simulink subsystem "FlightControl"  (R2024b)
settings: Solver=VariableStepAuto  StartTime=0.0  StopTime=10.0  RelTol=1e-3
undefined symbols (not defined in the file): control, controlParams, ControlSampleTime, CriticalTiltAngle, DiscIntNeverNeededParam, flightState, FWControlParams, FWTrimSpeed, tilt_max, tilt_trim, TiltScheduleRate, uavParam, w_trim, WindDownRate
libraries: slpidlib x31, simulink x9
(part 1 of 5)
settings Model: Creator=jjha  LastModifiedBy=jjha

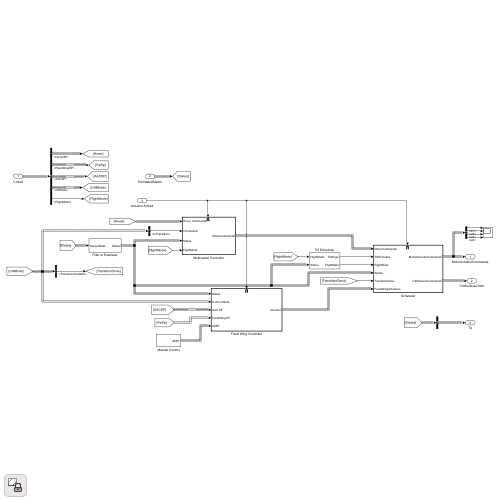
[thumbnail: Simulink's stored preview of the top-level diagram]
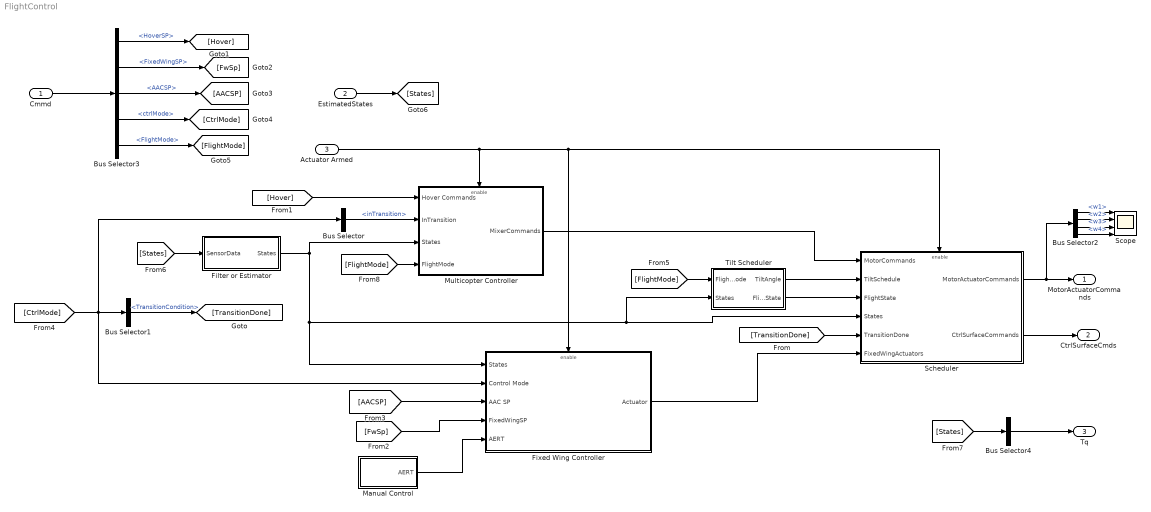
== system FlightControl ==
  Cmmd : Inport
  EstimatedStates : Inport  Port=2
  Actuator Armed : Inport  Port=3
  Bus Selector : BusSelector  OutputSignals=inTransition
  Bus Selector1 : BusSelector  OutputSignals=TransitionCondition
  Bus Selector2 : BusSelector  OutputSignals=w1,w2,w3,w4
  Bus Selector3 : BusSelector  OutputSignals=HoverSP,FixedWingSP,AACSP,ctrlMode,FlightMode
  Bus Selector4 : BusSelector  OutputSignals=RotorParameters.T1,RotorParameters.T2,RotorParameters.T3,RotorParameters.T4  OutputAsBus=on
  Filter or Estimator : Subsystem
  Fixed Wing Controller : Subsystem  TreatAsAtomicUnit=on  VariantControl=Fixed Wing Controller
  Manual Control : Subsystem
  Multicopter Controller : Subsystem
  Scheduler : Subsystem  SystemSampleTime=0.005
  Scope : Scope  NumInputPorts=4
  Tilt Scheduler : Subsystem
  MotorActuatorCommands : Outport
  CtrlSurfaceCmds : Outport  Port=2
  Tq : Outport  Port=3
  wires:
  Bus Selector3/2 -> [FwSp]  "<FixedWingSP>"
  Bus Selector3/1 -> [Hover]  "<HoverSP>"
  Bus Selector1/1 -> [TransitionDone]  "<TransitionCondition>"
  [Hover] -> Multicopter Controller/1(Hover Commands)
  Cmmd/1 -> Bus Selector3/1
  Bus Selector3/3 -> [AACSP]  "<AACSP>"
  Bus Selector2/4 -> Scope/4  "<w4>"
  Bus Selector3/5 -> [FlightMode]  "<FlightMode>"
  [FlightMode] -> Tilt Scheduler/1(FlightMode)
  [States] -> Bus Selector4/1
  Manual Control/1(AERT) -> Fixed Wing Controller/5(AERT)
  Tilt Scheduler/2(FlightState) -> Scheduler/3(FlightState)
  [AACSP] -> Fixed Wing Controller/3(AAC SP)
  Bus Selector3/4 -> [CtrlMode]  "<ctrlMode>"
  Multicopter Controller/1(MixerCommands) -> Scheduler/1(MotorCommands)
  Scheduler/2(CtrlSurfaceCommands) -> CtrlSurfaceCmds/1
  [CtrlMode] -> Bus Selector/1, Bus Selector1/1, Fixed Wing Controller/2(Control Mode)
  Bus Selector2/3 -> Scope/3  "<w3>"
  [FwSp] -> Fixed Wing Controller/4(FixedWingSP)
  [TransitionDone] -> Scheduler/5(TransitionDone)
  EstimatedStates/1 -> [States]
  Filter or Estimator/1(States) -> Tilt Scheduler/2(States), Scheduler/4(States), Fixed Wing Controller/1(States), Multicopter Controller/3(States)
  Bus Selector/1 -> Multicopter Controller/2(InTransition)  "<inTransition>"
  Tilt Scheduler/1(TiltAngle) -> Scheduler/2(TiltSchedule)
  Scheduler/1(MotorActuatorCommands) -> Bus Selector2/1, MotorActuatorCommands/1
  Bus Selector4/1 -> Tq/1
  [States] -> Filter or Estimator/1(SensorData)
  Fixed Wing Controller/1(Actuator) -> Scheduler/6(FixedWingActuators)
  Bus Selector2/1 -> Scope/1  "<w1>"
  Bus Selector2/2 -> Scope/2  "<w2>"
  [FlightMode] -> Multicopter Controller/4(FlightMode)
  Actuator Armed/1 -> Multicopter Controller/Enable, Scheduler/Enable, Fixed Wing Controller/Enable

== system FlightControl/Filter or Estimator ==
  SensorData : Inport
  States : Outport
  wires:
  SensorData/1 -> States/1

== system FlightControl/Fixed Wing Controller ==
  States : Inport
  Control Mode : Inport  Port=2
  AAC SP : Inport  Port=3
  FixedWingSP : Inport  Port=4
  AERT : Inport  Port=5
  Enable : EnablePort
  Fixed Wing Controller Module : Subsystem  Variant=on  VariantControl=TuningMode == 0
  Actuator : Outport
  wires:
  Fixed Wing Controller Module/1(Actuator) -> Actuator/1
  AERT/1 -> Fixed Wing Controller Module/5(AERT)
  FixedWingSP/1 -> Fixed Wing Controller Module/4(FixedWingSP)
  AAC SP/1 -> Fixed Wing Controller Module/3(AAC SP)
  Control Mode/1 -> Fixed Wing Controller Module/2(Control Mode)
  States/1 -> Fixed Wing Controller Module/1(States)

== system FlightControl/Manual Control ==
  Bus Creator : BusCreator  Inputs=4
  Constant{,1..3} (4 alike) : Constant  Value=0
  AERT : Outport
  wires:
  Constant/1 -> Bus Creator/1  "aileron"
  Constant1/1 -> Bus Creator/2  "throttle"
  Constant2/1 -> Bus Creator/3  "elevator"
  Constant3/1 -> Bus Creator/4  "rudder"
  Bus Creator/1 -> AERT/1

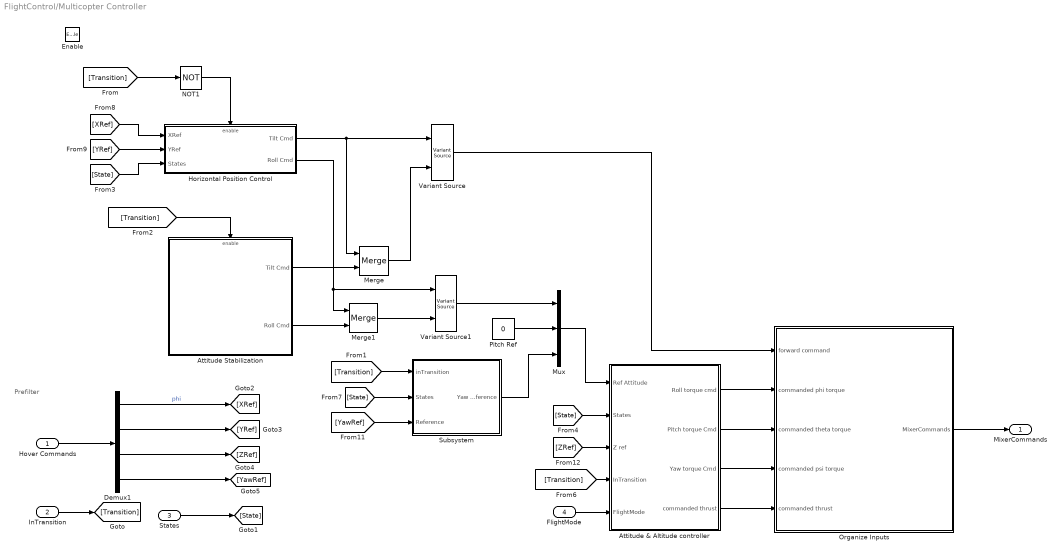
== system FlightControl/Multicopter Controller ==
  note: Prefilter
  Hover Commands : Inport
  InTransition : Inport  Port=2
  States : Inport  Port=3
  FlightMode : Inport  Port=4
  Enable : EnablePort
  Attitude & Altitude controller : Subsystem
  Attitude Stabilization : Subsystem  TreatAsAtomicUnit=on
  Demux1 : Demux
  Horizontal Position Control : Subsystem  TreatAsAtomicUnit=on
  Merge : Merge
  Merge1 : Merge
  Mux : Mux  Inputs=3
  NOT1 : Logic  Operator=NOT  IconShape=distinctive  AllPortsSameDT=off  OutDataTypeStr=boolean
  Organize Inputs : Subsystem
  Pitch Ref : Constant  Value=0
  Subsystem : Subsystem
  Variant Source : VariantSource
  Variant Source1 : VariantSource
  MixerCommands : Outport
  wires:
  Organize Inputs/1(MixerCommands) -> MixerCommands/1
  [Transition] -> Subsystem/1(inTransition)
  [State] -> Subsystem/2(States)
  Attitude Stabilization/2(Roll Cmd) -> Merge1/2
  Variant Source/1 -> Organize Inputs/1(forward command)
  [YawRef] -> Subsystem/3(Reference)
  Merge1/1 -> Variant Source1/2
  Horizontal Position Control/2(Roll Cmd) -> Merge1/1, Variant Source1/1
  Merge/1 -> Variant Source/2
  NOT1/1 -> Horizontal Position Control/Enable
  [Transition] -> Attitude Stabilization/Enable
  Pitch Ref/1 -> Mux/2
  [YRef] -> Horizontal Position Control/2(YRef)
  Attitude Stabilization/1(Tilt Cmd) -> Merge/2
  Demux1/3 -> [ZRef]
  [State] -> Attitude & Altitude controller/2(States)
  FlightMode/1 -> Attitude & Altitude controller/5(FlightMode)
  Attitude & Altitude controller/3(Yaw torque Cmd) -> Organize Inputs/4(commanded psi torque)
  [ZRef] -> Attitude & Altitude controller/3(Z ref)
  [XRef] -> Horizontal Position Control/1(XRef)
  Attitude & Altitude controller/4(commanded thrust) -> Organize Inputs/5(commanded thrust)
  InTransition/1 -> [Transition]
  States/1 -> [State]
  Subsystem/1(Yaw Reference) -> Mux/3
  Demux1/1 -> [XRef]  "phi"
  Attitude & Altitude controller/1(Roll torque cmd) -> Organize Inputs/2(commanded phi torque)
  Attitude & Altitude controller/2(Pitch torque Cmd) -> Organize Inputs/3(commanded theta torque)
  Hover Commands/1 -> Demux1/1
  Demux1/4 -> [YawRef]
  [Transition] -> NOT1/1
  Variant Source1/1 -> Mux/1
  [State] -> Horizontal Position Control/3(States)
  Horizontal Position Control/1(Tilt Cmd) -> Variant Source/1, Merge/1
  Mux/1 -> Attitude & Altitude controller/1(Ref Attitude)
  [Transition] -> Attitude & Altitude controller/4(InTransition)
  Demux1/2 -> [YRef]

== system FlightControl/Scheduler ==
  MotorCommands : Inport
  TiltSchedule : Inport  Port=2
  FlightState : Inport  Port=3  OutDataTypeStr=Enum: flightState
  States : Inport  Port=4
  TransitionDone : Inport  Port=5
  FixedWingActuators : Inport  Port=6
  Enable : EnablePort
  FixedWingScheduler : Subsystem
  MulticopterScheduler : Subsystem
  MotorActuatorCommands : Outport  OutputWhenDisabled=reset  InitialOutput=0
  CtrlSurfaceCommands : Outport  Port=2  OutDataTypeStr=Bus: FixedWingCtrlBus  OutputWhenDisabled=reset  InitialOutput=0  VectorParamsAs1DForOutWhenUnconnected=off
  wires:
  States/1 -> MulticopterScheduler/6(States)
  TransitionDone/1 -> FixedWingScheduler/3(TransitionDone), MulticopterScheduler/5(TransitionDone)
  FixedWingActuators/1 -> FixedWingScheduler/2(FixedWingActuators)
  MotorCommands/1 -> MulticopterScheduler/3(MotorCommands)
  MulticopterScheduler/1(ActuatorControls) -> MotorActuatorCommands/1
  TiltSchedule/1 -> MulticopterScheduler/4(TiltSchedule)
  FlightState/1 -> FixedWingScheduler/1(FlightState), MulticopterScheduler/1(FlightState)
  FixedWingScheduler/1(ActuatorControls) -> CtrlSurfaceCommands/1, MulticopterScheduler/2(FixedWingActuators)

== system FlightControl/Tilt Scheduler ==
  note: Back Transition Tilt Mode Manager
  note: Forward Transition Tilt Mode Manager
  FlightMode : Inport
  States : Inport  Port=2
  Back Transition Scheduler : Subsystem
  Forward Transition Scheduler : Subsystem
  TiltAngle : Outport
  FlightState : Outport  Port=2
  wires:
  Forward Transition Scheduler/2(Tilt Schedule) -> Back Transition Scheduler/1(Tilt Schedule)
  Forward Transition Scheduler/1(FlightState) -> FlightState/1
  FlightMode/1 -> Forward Transition Scheduler/1(FlightMode), Back Transition Scheduler/2(FlightMode)
  Back Transition Scheduler/1(TiltAngle) -> TiltAngle/1
  States/1 -> Back Transition Scheduler/3(States)

== system FlightControl/Fixed Wing Controller/Fixed Wing Controller Module ==
  States : Inport
  Control Mode : Inport  Port=2
  AAC SP : Inport  Port=3
  FixedWingSP : Inport  Port=4
  AERT : Inport  Port=5
  Fixed Wing Controller Simulation : Subsystem  VariantControl=TuningMode == 0
  Fixed Wing Controller Tuning : Subsystem  VariantControl=TuningMode==1
  Actuator : Outport

== system FlightControl/Multicopter Controller/Attitude & Altitude controller ==
  Ref Attitude : Inport
  States : Inport  Port=2
  Z ref : Inport  Port=3
  InTransition : Inport  Port=4
  FlightMode : Inport  Port=5
  Altitude Control : Subsystem
  Derivative Gain : Subsystem  VariantControl=AttitudeControl==1
  Roll torque cmd : Outport
  Pitch torque Cmd : Outport  Port=2
  Yaw torque Cmd : Outport  Port=3
  commanded thrust : Outport  Port=4
  wires:
  Ref Attitude/1 -> Derivative Gain/1(Ref Attitude)
  FlightMode/1 -> Altitude Control/4(FlightMode)
  Z ref/1 -> Altitude Control/2(Z ref)
  Derivative Gain/3(Yaw torque Cmd) -> Yaw torque Cmd/1
  States/1 -> Derivative Gain/2(States), Altitude Control/1(States)
  Derivative Gain/2(Pitch torque Cmd) -> Pitch torque Cmd/1
  InTransition/1 -> Altitude Control/3(InTransition)
  Derivative Gain/1(Roll torque cmd) -> Roll torque cmd/1
  Altitude Control/1(commanded thrust) -> commanded thrust/1

== system FlightControl/Multicopter Controller/Attitude Stabilization ==
  note: Level Tiltrotor when in transition.
  Enable : EnablePort
  Constant : Constant  Value=0
  Constant1 : Constant  Value=0
  Tilt Cmd : Outport
  Roll Cmd : Outport  Port=2
  wires:
  Constant1/1 -> Roll Cmd/1
  Constant/1 -> Tilt Cmd/1

== system FlightControl/Multicopter Controller/Horizontal Position Control ==
  note: Forward Motion is controlled using Tilt.
      | Lateral Motion occurs using roll.
  XRef : Inport
  YRef : Inport  Port=2
  States : Inport  Port=3
  Enable : EnablePort
  Rate Limiter : RateLimiter  RisingSlewLimit=5.1  FallingSlewLimit=-5.1  SampleTimeMode=inherited
  Saturation : Saturate  UpperLimit=0.25  LowerLimit=-0.25
  Saturation1 : Saturate  UpperLimit=0.75  LowerLimit=-0.75
  XY Controller : Subsystem
  Tilt Cmd : Outport
  Roll Cmd : Outport  Port=2
  wires:
  Rate Limiter/1 -> Roll Cmd/1
  Saturation/1 -> Rate Limiter/1
  Saturation1/1 -> Tilt Cmd/1
  XY Controller/2(Sideward Cmd) -> Saturation/1
  XY Controller/1(Forward cmd) -> Saturation1/1
  States/1 -> XY Controller/3(States)
  YRef/1 -> XY Controller/2(Y_ref)
  XRef/1 -> XY Controller/1(X_ref)

== system FlightControl/Multicopter Controller/Organize Inputs ==
  forward command : Inport
  commanded phi torque : Inport  Port=2
  commanded theta torque : Inport  Port=3
  commanded psi torque : Inport  Port=4
  commanded thrust : Inport  Port=5
  Out Bus Element : Outport  PortName=MixerCommands  Element=w_phi
  Out Bus Element1 : Outport  PortName=MixerCommands  Element=w_theta
  Out Bus Element2 : Outport  PortName=MixerCommands  Element=l_psi
  Out Bus Element3 : Outport  PortName=MixerCommands  Element=w_z
  Out Bus Element4 : Outport  PortName=MixerCommands  Element=l_x
  tag scope: w_phi=global, w_psi=global, w_theta=global, w_tilt=global, w_z=global
  wires:
  commanded phi torque/1 -> Out Bus Element/1, [w_phi]  "phi"
  forward command/1 -> Out Bus Element4/1, [w_tilt]
  commanded thrust/1 -> Out Bus Element3/1, [w_z]
  commanded psi torque/1 -> Out Bus Element2/1, [w_psi]
  commanded theta torque/1 -> Out Bus Element1/1, [w_theta]  "theta"

== system FlightControl/Multicopter Controller/Subsystem ==
  inTransition : Inport
  States : Inport  Port=2
  Reference : Inport  Port=3
  Bus Selector : BusSelector  OutputSignals=ypr
  NOT : Logic  Operator=NOT  IconShape=distinctive  AllPortsSameDT=off  OutDataTypeStr=boolean
  Selector : Selector  InputPortWidth=3  IndexOptions=Index vector (dialog)  Indices=[1]  OutputSizes=1
  Switch : Switch  Criteria=u2 > Threshold  SaturateOnIntegerOverflow=off  InputSameDT=off
  Triggered Subsystem : Subsystem  TreatAsAtomicUnit=on
  Yaw Reference : Outport
  wires:
  Reference/1 -> Switch/1
  Switch/1 -> Yaw Reference/1
  Triggered Subsystem/1(Reference) -> Switch/3  "Stable"
  NOT/1 -> Switch/2
  Selector/1 -> Triggered Subsystem/1(YawHold)
  Bus Selector/1 -> Selector/1  "<ypr>"
  States/1 -> Bus Selector/1
  inTransition/1 -> NOT/1, Triggered Subsystem/Trigger

== system FlightControl/Scheduler/FixedWingScheduler ==
  note: Fixed Wing Control Mixer
  note: C opyright 2024 The MathWorks, Inc.
  FlightState : Inport
  FixedWingActuators : Inport  Port=2  OutDataTypeStr=Bus: FixedWingCtrlBus
  TransitionDone : Inport  Port=3
  Merge : Merge  Inputs=4
  Switch Case : SwitchCase  CaseConditions={flightState.Hover, flightState.Transition, flightState.FixedWing,flightState.BackTransition}  ShowDefaultCase=off
  Switch Case Action Subsystem : Subsystem  TreatAsAtomicUnit=on
  Switch Case Action Subsystem1 : Subsystem  TreatAsAtomicUnit=on
  Switch Case Action Subsystem2 : Subsystem  TreatAsAtomicUnit=on
  Switch Case Action Subsystem3 : Subsystem  TreatAsAtomicUnit=on
  ActuatorControls : Outport
  wires:
  Switch Case Action Subsystem2/1(FixedWingControls) -> Merge/3
  Switch Case/1 -> Switch Case Action Subsystem/Action
  Switch Case Action Subsystem/1(FixedWingControls) -> Merge/1
  Switch Case/4 -> Switch Case Action Subsystem3/Action
  Switch Case Action Subsystem1/1(FixedWingControls) -> Merge/2
  Merge/1 -> ActuatorControls/1
  Switch Case Action Subsystem3/1(FixedWingControls) -> Merge/4
  TransitionDone/1 -> Switch Case Action Subsystem1/2(TransitionDone)
  Switch Case/2 -> Switch Case Action Subsystem1/Action
  Switch Case/3 -> Switch Case Action Subsystem2/Action
  FixedWingActuators/1 -> Switch Case Action Subsystem1/1(FixedWingActuators), Switch Case Action Subsystem2/1(FixedWingActuators)
  FlightState/1 -> Switch Case/1

== system FlightControl/Scheduler/MulticopterScheduler ==
  note: Multicopter Control Mixer
  note: C opyright 2024 The MathWorks, Inc.
  FlightState : Inport
  FixedWingActuators : Inport  Port=2
  MotorCommands : Inport  Port=3
  TiltSchedule : Inport  Port=4
  TransitionDone : Inport  Port=5
  States : Inport  Port=6
  Actuator To Voltage : Subsystem
  Merge : Merge  Inputs=4
  Switch Case : SwitchCase  CaseConditions={flightState.Hover, flightState.Transition, flightState.FixedWing,flightState.BackTransition}  ShowDefaultCase=off
  Switch Case Action Subsystem : Subsystem  TreatAsAtomicUnit=on
  Switch Case Action Subsystem1 : Subsystem  TreatAsAtomicUnit=on
  Switch Case Action Subsystem2 : Subsystem  TreatAsAtomicUnit=on
  Switch Case Action Subsystem3 : Subsystem  TreatAsAtomicUnit=on
  ActuatorControls : Outport  OutDataTypeStr=Bus: RotorCntrlBus
  wires:
  Switch Case/1 -> Switch Case Action Subsystem/Action
  TiltSchedule/1 -> Switch Case Action Subsystem3/2(TiltSchedule), Switch Case Action Subsystem1/1(TiltSchedule)
  Switch Case Action Subsystem1/1(Actuator) -> Merge/2
  Switch Case/2 -> Switch Case Action Subsystem1/Action
  Actuator To Voltage/1(To PWM) -> ActuatorControls/1
  TransitionDone/1 -> Switch Case Action Subsystem1/4(TransitionDone), Switch Case Action Subsystem2/2(TransitionDone)
  Switch Case/3 -> Switch Case Action Subsystem2/Action
  FixedWingActuators/1 -> Switch Case Action Subsystem2/1(FixedWingCtrlBus), Switch Case Action Subsystem1/3(FixedWing)
  Switch Case Action Subsystem3/1(Actuator) -> Merge/4
  Switch Case Action Subsystem/1(Actuator) -> Merge/1
  FlightState/1 -> Switch Case/1
  Switch Case Action Subsystem2/1(Actuator) -> Merge/3
  States/1 -> Switch Case Action Subsystem1/5(State), Switch Case Action Subsystem2/3(State)
  MotorCommands/1 -> Switch Case Action Subsystem3/1(MixerCommands), Switch Case Action Subsystem1/2(MixerCommands), Switch Case Action Subsystem/1(MixerCommands)
  Switch Case/4 -> Switch Case Action Subsystem3/Action
  Merge/1 -> Actuator To Voltage/1(Motor Commands)

== system FlightControl/Tilt Scheduler/Back Transition Scheduler ==
  Tilt Schedule : Inport
  FlightMode : Inport  Port=2
  States : Inport  Port=3
  Add : Sum  Inputs=+-
  Bus Selector : BusSelector  OutputSignals=Vb
  Constant1 : Constant  Value=flightState.BackTransition
  Constant6 : Constant  Value=4
  Equal1 : RelationalOperator  Operator===  OutDataTypeStr=boolean  RndMeth=Simplest  InputSameDT=off
  Saturation : Saturate  UpperLimit=pi/4  LowerLimit=-pi/4
  Selector : Selector  InputPortWidth=3  IndexOptions=Index vector (dialog)  Indices=[1]  OutputSizes=1
  Switch2 : Switch  Threshold=1  SaturateOnIntegerOverflow=off  InputSameDT=off
  Vx Controller : slpidlib/PID Controller  Controller=P  Form=Parallel  TimeDomain=Discrete-time  UseExternalTs=off  SampleTime=0.005  IntegratorMethod=Forward Euler  FilterMethod=Forward Euler  ControllerParametersSource=internal  P=controlParams.P_BACK  I=0  UseKiTs=off  D=0.0379422021775223  UseExternalDerivativeSource=off  N=1.96946409823213  UseFilter=on  TunerSelectOption=Transfer Function Based (PID Tuner App)  InitialConditionSource=internal  InitialConditionForIntegrator=0  InitialConditionForFilter=0  DifferentiatorICPrevScaledInput=0  ExternalReset=none  TrackingMode=off  Kt=1  LimitOutput=off  SatLimitsSource=internal  UpperSaturationLimit=inf  LowerSaturationLimit=-inf  LinearizeAsGain=on  AntiWindupMode=none  Kb=1  LimitIntegrator=off  UpperIntegratorSaturationLimit=inf  LowerIntegratorSaturationLimit=-inf  POutMin=[]  POutMax=[]  IOutMin=[]  IOutMax=[]  DOutMin=[]  DOutMax=[]  NOutMin=[]  NOutMax=[]  SumOutMin=[]  SumOutMax=[]  SaturationOutMin=[]  SaturationOutMax=[]  PParamMin=[]  PParamMax=[]  IParamMin=[]  IParamMax=[]  DParamMin=[]  DParamMax=[]  NParamMin=[]  NParamMax=[]  KbParamMin=[]  KbParamMax=[]  KtParamMin=[]  KtParamMax=[]  KbOutMin=[]  KbOutMax=[]  KtOutMin=[]  KtOutMax=[]  IntegratorOutMin=[]  IntegratorOutMax=[]  FilterOutMin=[]  FilterOutMax=[]  SumI1OutMin=[]  SumI1OutMax=[]  SumI2OutMin=[]  SumI2OutMax=[]  SumI3OutMin=[]  SumI3OutMax=[]  SumI4OutMin=[]  SumI4OutMax=[]  SumDOutMin=[]  SumDOutMax=[]  DifferentiatorOutMin=[]  DifferentiatorOutMax=[]  FilterDiffOutCoefMin=[]  FilterDiffOutCoefMax=[]  ReciprocalOutMin=[]  ReciprocalOutMax=[]  SumDenOutMin=[]  SumDenOutMax=[]  SumNumOutMin=[]  SumNumOutMax=[]  DivideOutMin=[]  DivideOutMax=[]  UdiffTsProdOutMin=[]  UdiffTsProdOutMax=[]  NTsProdOutMin=[]  NTsProdOutMax=[]  UintegralTsProdOutMin=[]  UintegralTsProdOutMax=[]  UngainTsProdOutMin=[]  UngainTsProdOutMax=[]  ClampingZeroOutDataTypeStr=Inherit: Inherit via back propagation  ClampingZeroOutMin=[]  ClampingZeroOutMax=[]  FilterDenConstantOutDataTypeStr=Inherit: Inherit via back propagation  FilterDenConstantOutMin=[]  FilterDenConstantOutMax=[]  PCopyOutDataTypeStr=Inherit: Inherit via back propagation  PCopyOutMin=[]  PCopyOutMax=[]  NCopyOutDataTypeStr=Inherit: Inherit via back propagation  NCopyOutMin=[]  NCopyOutMax=[]  IntegratorContinuousStateAttributes=''  IntegratorStateMustResolveToSignalObject=off  IntegratorRTWStateStorageClass=Auto  FilterContinuousStateAttributes=''  FilterStateMustResolveToSignalObject=off  FilterRTWStateStorageClass=Auto  ParallelPVariant=InternalParameters  IdealPVariant=Disabled  IVariant=Disabled  DVariant=Disabled  IntegratorVariant=Disabled  SatVariant=Disabled  AWVariant=Disabled  PCopyVariant=Disabled  TRVariant=Disabled  FdbkBlocksVariant=Forward  IdealPFdbkVariant=Disabled  SatFdbkVariant=Disabled  DerivativeFilterVariant=Disabled  NVariant=Disabled  NCopyVariant=Disabled_SignalSpec  FilterICVariant=Disabled  IntegratorICVariant=Disabled  ExternalResetVariant=Disabled  TRSumVariant=Passthrough  SumFdbkVariant=Disabled  SumVariant=Passthrough_P  TsampFilterVariant=InternalTs  TsampNgainVariant=Passthrough  TsampIntegralVariant=Disabled_SignalSpec  ExternalSaturationOutDataTypeStr=Inherit: Same as second input  DerivativeSourceVariant=Disabled  PreIntVariant=InternalPreInt
  TiltAngle : Outport
  wires:
  Switch2/1 -> TiltAngle/1
  Tilt Schedule/1 -> Switch2/3
  Saturation/1 -> Switch2/1
  Vx Controller/1 -> Saturation/1
  Selector/1 -> Add/2
  Constant6/1 -> Add/1
  Constant1/1 -> Equal1/2
  FlightMode/1 -> Equal1/1
  Bus Selector/1 -> Selector/1  "<Vb>"
  Equal1/1 -> Switch2/2
  Add/1 -> Vx Controller/1
  States/1 -> Bus Selector/1

== system FlightControl/Tilt Scheduler/Forward Transition Scheduler ==
  FlightMode : Inport
  Constant : Constant  Value=pi/2
  Constant2 : Constant  Value=0
  Constant3 : Constant  Value=CriticalTiltAngle
  Constant4 : Constant  Value=flightState.Transition
  Constant5 : Constant  Value=TiltScheduleRate
  Discrete-Time Integrator : DiscreteIntegrator  ExternalReset=either  SampleTime=-1  LimitOutput=on  LowerSaturationLimit=0  ICPrevOutput=DiscIntNeverNeededParam  ICPrevScaledInput=DiscIntNeverNeededParam
  Equal : RelationalOperator  Operator===  OutDataTypeStr=boolean  RndMeth=Simplest  InputSameDT=off
  LessThanOrEqual : RelationalOperator  Operator=<=  OutDataTypeStr=boolean  RndMeth=Simplest  InputSameDT=off
  Switch : Switch  Criteria=u2 > Threshold  SaturateOnIntegerOverflow=off  InputSameDT=off
  Switch1 : Switch  Criteria=u2 > Threshold  SaturateOnIntegerOverflow=off  InputSameDT=off
  FlightState : Outport
  Tilt Schedule : Outport  Port=2
  tag scope: ModeFlag=global
  wires:
  Switch/1 -> Tilt Schedule/1
  Constant/1 -> Switch/3
  Constant4/1 -> Equal/1
  Constant2/1 -> Switch1/3
  Constant5/1 -> Switch1/1
  Switch1/1 -> Discrete-Time Integrator/1
  Constant3/1 -> LessThanOrEqual/2
  Equal/1 -> [ModeFlag]
  LessThanOrEqual/1 -> Switch/2
  Discrete-Time Integrator/1 -> Switch/1, LessThanOrEqual/1
  [ModeFlag] -> Switch1/2, Discrete-Time Integrator/2
  FlightMode/1 -> Equal/2, FlightState/1

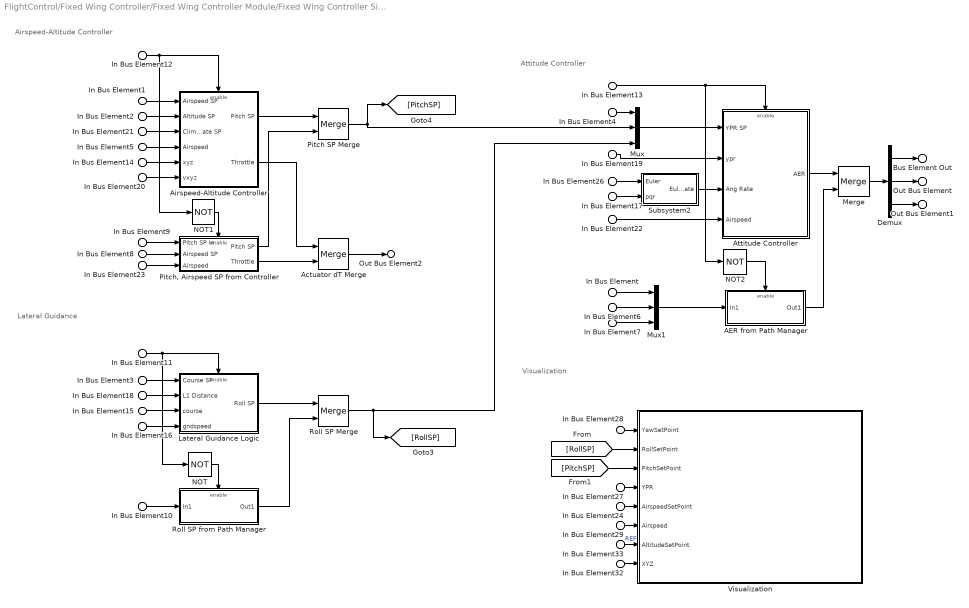
== system FlightControl/Fixed Wing Controller/Fixed Wing Controller Module/Fixed Wing Controller Simulation ==
  note: Visualization
  note: Airspeed-Altitude Controller
  note: Lateral Guidance
  note: Attitude Controller
  In Bus Element14 : Inport  PortName=States  Element=Xe
  In Bus Element32 : Inport  PortName=States  Element=Xe
  In Bus Element15 : Inport  PortName=States  Element=course
  In Bus Element17 : Inport  PortName=States  Element=pqr
  In Bus Element{5,22..23,29} (4 alike) : Inport  PortName=States  Element=airspeed
  In Bus Element19 : Inport  PortName=States  Element=ypr
  In Bus Element27 : Inport  PortName=States  Element=ypr
  In Bus Element16 : Inport  PortName=States  Element=gndspeed
  In Bus Element26 : Inport  PortName=States  Element=Euler
  In Bus Element20 : Inport  PortName=States  Element=Ve_ground
  In Bus Element11 : Inport  Port=2  PortName=Control Mode  Element=lateralGuidance
  In Bus Element12 : Inport  Port=2  PortName=Control Mode  Element=airspeedAltitude
  In Bus Element13 : Inport  Port=2  PortName=Control Mode  Element=attitude
  In Bus Element1 : Inport  Port=3  PortName=AAC SP  Element=airspeed
  In Bus Element24 : Inport  Port=3  PortName=AAC SP  Element=airspeed
  In Bus Element2 : Inport  Port=3  PortName=AAC SP  Element=altitude
  In Bus Element33 : Inport  Port=3  PortName=AAC SP  Element=altitude
  In Bus Element18 : Inport  Port=3  PortName=AAC SP  Element=L1
  In Bus Element21 : Inport  Port=3  PortName=AAC SP  Element=course
  In Bus Element3 : Inport  Port=3  PortName=AAC SP  Element=course
  In Bus Element4 : Inport  Port=4  PortName=FixedWingSP  Element=yaw
  In Bus Element28 : Inport  Port=4  PortName=FixedWingSP  Element=yaw
  In Bus Element9 : Inport  Port=4  PortName=FixedWingSP  Element=pitch
  In Bus Element10 : Inport  Port=4  PortName=FixedWingSP  Element=roll
  In Bus Element8 : Inport  Port=4  PortName=FixedWingSP  Element=airspeed
  In Bus Element : Inport  Port=5  PortName=AERT  Element=aileron
  In Bus Element6 : Inport  Port=5  PortName=AERT  Element=elevator
  In Bus Element7 : Inport  Port=5  PortName=AERT  Element=rudder
  AER from Path Manager : Subsystem  TreatAsAtomicUnit=on
  Actuator dT Merge : Merge
  Airspeed-Altitude Controller : Subsystem
  Attitude Controller : Subsystem
  Demux : Demux  Outputs=3
  Lateral Guidance Logic : Subsystem
  Merge : Merge
  Mux : Mux  Inputs=3
  Mux1 : Mux  Inputs=3
  NOT : Logic  Operator=NOT  IconShape=distinctive  AllPortsSameDT=off  OutDataTypeStr=boolean
  NOT1 : Logic  Operator=NOT  IconShape=distinctive  AllPortsSameDT=off  OutDataTypeStr=boolean
  NOT2 : Logic  Operator=NOT  IconShape=distinctive  AllPortsSameDT=off  OutDataTypeStr=boolean
  Pitch SP Merge : Merge
  "Pitch, Airspeed SP from Controller" : Subsystem  TreatAsAtomicUnit=on
  Roll SP Merge : Merge
  Roll SP from Path Manager : Subsystem  TreatAsAtomicUnit=on
  Subsystem2 : Subsystem
  Visualization : Subsystem  Variant=on  VariantControl=Visualization
  Bus Element Out : Outport  PortName=Actuator  Element=dA
  Out Bus Element : Outport  PortName=Actuator  Element=dE
  Out Bus Element1 : Outport  PortName=Actuator  Element=dR
  Out Bus Element2 : Outport  PortName=Actuator  Element=dT
  wires:
  [PitchSP] -> Visualization/3(PitchSetPoint)
  [RollSP] -> Visualization/2(RollSetPoint)
  In Bus Element32/1 -> Visualization/8(XYZ)
  In Bus Element33/1 -> Visualization/7(AltitudeSetPoint)  "REF"
  In Bus Element29/1 -> Visualization/6(Airspeed)
  In Bus Element24/1 -> Visualization/5(AirspeedSetPoint)
  In Bus Element27/1 -> Visualization/4(YPR)
  In Bus Element28/1 -> Visualization/1(YawSetPoint)
  In Bus Element12/1 -> NOT1/1, Airspeed-Altitude Controller/Enable
  Roll SP Merge/1 -> Mux/3, [RollSP]
  In Bus Element21/1 -> Airspeed-Altitude Controller/3(Climb Rate SP)
  Demux/1 -> Bus Element Out/1
  In Bus Element5/1 -> Airspeed-Altitude Controller/4(Airspeed)
  AER from Path Manager/1(Out1) -> Merge/2
  NOT/1 -> Roll SP from Path Manager/Enable
  Lateral Guidance Logic/1(Roll SP) -> Roll SP Merge/1
  In Bus Element23/1 -> "Pitch, Airspeed SP from Controller"/3(Airspeed)
  NOT2/1 -> AER from Path Manager/Enable
  In Bus Element19/1 -> Attitude Controller/2(ypr)
  In Bus Element20/1 -> Airspeed-Altitude Controller/6(vxyz)
  In Bus Element8/1 -> "Pitch, Airspeed SP from Controller"/2(Airspeed SP)
  NOT1/1 -> "Pitch, Airspeed SP from Controller"/Enable
  Attitude Controller/1(AER) -> Merge/1
  Mux/1 -> Attitude Controller/1(YPR SP)
  In Bus Element10/1 -> Roll SP from Path Manager/1(In1)
  Merge/1 -> Demux/1
  In Bus Element9/1 -> "Pitch, Airspeed SP from Controller"/1(Pitch SP In)
  In Bus Element7/1 -> Mux1/3
  In Bus Element2/1 -> Airspeed-Altitude Controller/2(Altitude SP)
  In Bus Element/1 -> Mux1/1
  "Pitch, Airspeed SP from Controller"/2(Throttle) -> Actuator dT Merge/2
  In Bus Element16/1 -> Lateral Guidance Logic/4(gndspeed)
  "Pitch, Airspeed SP from Controller"/1(Pitch SP) -> Pitch SP Merge/2
  Airspeed-Altitude Controller/2(Throttle) -> Actuator dT Merge/1
  Mux1/1 -> AER from Path Manager/1(In1)
  In Bus Element6/1 -> Mux1/2
  In Bus Element15/1 -> Lateral Guidance Logic/3(course)
  In Bus Element14/1 -> Airspeed-Altitude Controller/5(xyz)
  In Bus Element4/1 -> Mux/1
  Roll SP from Path Manager/1(Out1) -> Roll SP Merge/2
  Demux/3 -> Out Bus Element1/1
  In Bus Element22/1 -> Attitude Controller/4(Airspeed)
  In Bus Element3/1 -> Lateral Guidance Logic/1(Course SP)
  In Bus Element13/1 -> Attitude Controller/Enable, NOT2/1
  Subsystem2/1(Euler Rate) -> Attitude Controller/3(Ang Rate)
  In Bus Element11/1 -> NOT/1, Lateral Guidance Logic/Enable
  In Bus Element26/1 -> Subsystem2/1(Euler)
  Actuator dT Merge/1 -> Out Bus Element2/1
  In Bus Element17/1 -> Subsystem2/2(pqr)
  In Bus Element1/1 -> Airspeed-Altitude Controller/1(Airspeed SP)
  In Bus Element18/1 -> Lateral Guidance Logic/2(L1 Distance)
  Airspeed-Altitude Controller/1(Pitch SP) -> Pitch SP Merge/1
  Demux/2 -> Out Bus Element/1
  Pitch SP Merge/1 -> [PitchSP], Mux/2

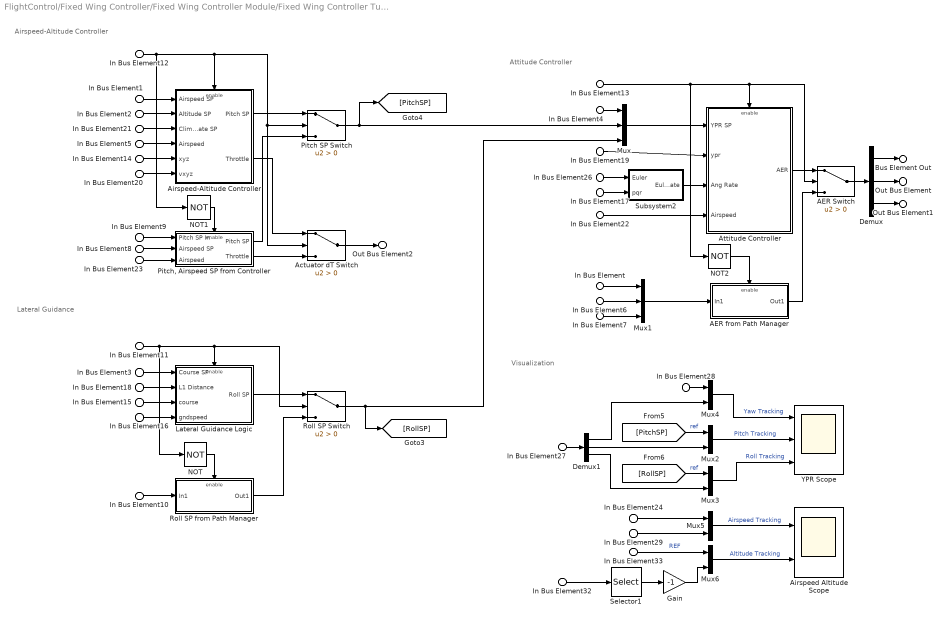
== system FlightControl/Fixed Wing Controller/Fixed Wing Controller Module/Fixed Wing Controller Tuning ==
  note: Lateral Guidance
  note: Airspeed-Altitude Controller
  note: Attitude Controller
  note: Visualization
  In Bus Element14 : Inport  PortName=States  Element=Xe
  In Bus Element32 : Inport  PortName=States  Element=Xe
  In Bus Element15 : Inport  PortName=States  Element=course
  In Bus Element17 : Inport  PortName=States  Element=pqr
  In Bus Element{5,22..23,29} (4 alike) : Inport  PortName=States  Element=airspeed
  In Bus Element19 : Inport  PortName=States  Element=ypr
  In Bus Element27 : Inport  PortName=States  Element=ypr
  In Bus Element16 : Inport  PortName=States  Element=gndspeed
  In Bus Element26 : Inport  PortName=States  Element=Euler
  In Bus Element20 : Inport  PortName=States  Element=Ve_ground
  In Bus Element11 : Inport  Port=2  PortName=Control Mode  Element=lateralGuidance
  In Bus Element12 : Inport  Port=2  PortName=Control Mode  Element=airspeedAltitude
  In Bus Element13 : Inport  Port=2  PortName=Control Mode  Element=attitude
  In Bus Element1 : Inport  Port=3  PortName=AAC SP  Element=airspeed
  In Bus Element24 : Inport  Port=3  PortName=AAC SP  Element=airspeed
  In Bus Element2 : Inport  Port=3  PortName=AAC SP  Element=altitude
  In Bus Element33 : Inport  Port=3  PortName=AAC SP  Element=altitude
  In Bus Element18 : Inport  Port=3  PortName=AAC SP  Element=L1
  In Bus Element21 : Inport  Port=3  PortName=AAC SP  Element=course
  In Bus Element3 : Inport  Port=3  PortName=AAC SP  Element=course
  In Bus Element4 : Inport  Port=4  PortName=FixedWingSP  Element=yaw
  In Bus Element28 : Inport  Port=4  PortName=FixedWingSP  Element=yaw
  In Bus Element9 : Inport  Port=4  PortName=FixedWingSP  Element=pitch
  In Bus Element10 : Inport  Port=4  PortName=FixedWingSP  Element=roll
  In Bus Element8 : Inport  Port=4  PortName=FixedWingSP  Element=airspeed
  In Bus Element : Inport  Port=5  PortName=AERT  Element=aileron
  In Bus Element6 : Inport  Port=5  PortName=AERT  Element=elevator
  In Bus Element7 : Inport  Port=5  PortName=AERT  Element=rudder
  AER Switch : Switch  Criteria=u2 > Threshold  SaturateOnIntegerOverflow=off  InputSameDT=off
  AER from Path Manager : Subsystem  TreatAsAtomicUnit=on
  Actuator dT Switch : Switch  Criteria=u2 > Threshold  SaturateOnIntegerOverflow=off  InputSameDT=off
  Airspeed Altitude Scope : Scope  NumInputPorts=2
  Airspeed-Altitude Controller : Subsystem
  Attitude Controller : Subsystem
  Demux : Demux  Outputs=3
  Demux1 : Demux  Outputs=3
  Gain : Gain  Gain=-1
  Lateral Guidance Logic : Subsystem
  Mux : Mux  Inputs=3
  Mux1 : Mux  Inputs=3
  Mux{2..6} (5 alike) : Mux  Inputs=2
  NOT : Logic  Operator=NOT  IconShape=distinctive  AllPortsSameDT=off  OutDataTypeStr=boolean
  NOT1 : Logic  Operator=NOT  IconShape=distinctive  AllPortsSameDT=off  OutDataTypeStr=boolean
  NOT2 : Logic  Operator=NOT  IconShape=distinctive  AllPortsSameDT=off  OutDataTypeStr=boolean
  Pitch SP Switch : Switch  Criteria=u2 > Threshold  SaturateOnIntegerOverflow=off  InputSameDT=off
  "Pitch, Airspeed SP from Controller" : Subsystem  TreatAsAtomicUnit=on
  Roll SP Switch : Switch  Criteria=u2 > Threshold  SaturateOnIntegerOverflow=off  InputSameDT=off
  Roll SP from Path Manager : Subsystem  TreatAsAtomicUnit=on
  Selector1 : Selector  InputPortWidth=3  IndexOptions=Index vector (dialog)  Indices=[3]  OutputSizes=1
  Subsystem2 : Subsystem
  YPR Scope : Scope  NumInputPorts=3
  Bus Element Out : Outport  PortName=Actuator  Element=dA
  Out Bus Element : Outport  PortName=Actuator  Element=dE
  Out Bus Element1 : Outport  PortName=Actuator  Element=dR
  Out Bus Element2 : Outport  PortName=Actuator  Element=dT
  wires:
  In Bus Element33/1 -> Mux6/1  "REF"
  Gain/1 -> Mux6/2
  Selector1/1 -> Gain/1
  In Bus Element32/1 -> Selector1/1
  In Bus Element29/1 -> Mux5/2
  In Bus Element24/1 -> Mux5/1
  Mux6/1 -> Airspeed Altitude Scope/2  "Altitude Tracking"
  Mux5/1 -> Airspeed Altitude Scope/1  "Airspeed Tracking"
  Mux3/1 -> YPR Scope/3  "Roll Tracking"
  Mux2/1 -> YPR Scope/2  "Pitch Tracking"
  Mux4/1 -> YPR Scope/1  "Yaw Tracking"
  [RollSP] -> Mux3/1  "ref"
  In Bus Element28/1 -> Mux4/1
  [PitchSP] -> Mux2/1  "ref"
  Airspeed-Altitude Controller/1(Pitch SP) -> Pitch SP Switch/1
  Pitch SP Switch/1 -> Mux/2, [PitchSP]
  Demux/2 -> Out Bus Element/1
  Actuator dT Switch/1 -> Out Bus Element2/1
  Subsystem2/1(Euler Rate) -> Attitude Controller/3(Ang Rate)
  In Bus Element26/1 -> Subsystem2/1(Euler)
  In Bus Element17/1 -> Subsystem2/2(pqr)
  Demux1/3 -> Mux3/2
  Demux1/2 -> Mux2/2
  Demux1/1 -> Mux4/2
  In Bus Element27/1 -> Demux1/1
  In Bus Element23/1 -> "Pitch, Airspeed SP from Controller"/3(Airspeed)
  In Bus Element21/1 -> Airspeed-Altitude Controller/3(Climb Rate SP)
  In Bus Element20/1 -> Airspeed-Altitude Controller/6(vxyz)
  In Bus Element1/1 -> Airspeed-Altitude Controller/1(Airspeed SP)
  In Bus Element3/1 -> Lateral Guidance Logic/1(Course SP)
  In Bus Element22/1 -> Attitude Controller/4(Airspeed)
  In Bus Element4/1 -> Mux/1
  In Bus Element13/1 -> Attitude Controller/Enable, AER Switch/2, NOT2/1
  Demux/3 -> Out Bus Element1/1
  In Bus Element15/1 -> Lateral Guidance Logic/3(course)
  Roll SP Switch/1 -> [RollSP], Mux/3
  In Bus Element2/1 -> Airspeed-Altitude Controller/2(Altitude SP)
  In Bus Element12/1 -> NOT1/1, Airspeed-Altitude Controller/Enable, Pitch SP Switch/2, Actuator dT Switch/2
  In Bus Element5/1 -> Airspeed-Altitude Controller/4(Airspeed)
  In Bus Element16/1 -> Lateral Guidance Logic/4(gndspeed)
  In Bus Element19/1 -> Attitude Controller/2(ypr)
  In Bus Element14/1 -> Airspeed-Altitude Controller/5(xyz)
  In Bus Element18/1 -> Lateral Guidance Logic/2(L1 Distance)
  In Bus Element11/1 -> NOT/1, Lateral Guidance Logic/Enable, Roll SP Switch/2
  In Bus Element10/1 -> Roll SP from Path Manager/1(In1)
  In Bus Element9/1 -> "Pitch, Airspeed SP from Controller"/1(Pitch SP In)
  In Bus Element7/1 -> Mux1/3
  In Bus Element6/1 -> Mux1/2
  In Bus Element/1 -> Mux1/1
  NOT2/1 -> AER from Path Manager/Enable
  AER from Path Manager/1(Out1) -> AER Switch/3
  Mux1/1 -> AER from Path Manager/1(In1)
  "Pitch, Airspeed SP from Controller"/2(Throttle) -> Actuator dT Switch/3
  Airspeed-Altitude Controller/2(Throttle) -> Actuator dT Switch/1
  "Pitch, Airspeed SP from Controller"/1(Pitch SP) -> Pitch SP Switch/3
  In Bus Element8/1 -> "Pitch, Airspeed SP from Controller"/2(Airspeed SP)
  NOT1/1 -> "Pitch, Airspeed SP from Controller"/Enable
  Roll SP from Path Manager/1(Out1) -> Roll SP Switch/3
  Lateral Guidance Logic/1(Roll SP) -> Roll SP Switch/1
  NOT/1 -> Roll SP from Path Manager/Enable
  Demux/1 -> Bus Element Out/1
  AER Switch/1 -> Demux/1
  Attitude Controller/1(AER) -> AER Switch/1
  Mux/1 -> Attitude Controller/1(YPR SP)

== system FlightControl/Multicopter Controller/Attitude & Altitude controller/Altitude Control ==
  note: Maintain altitude previously set when in transition
  States : Inport
  Z ref : Inport  Port=2
  InTransition : Inport  Port=3
  FlightMode : Inport  Port=4
  Alt signal condition : Subsystem
  Altitude controller : slpidlib/PID Controller  Controller=P  Form=Parallel  TimeDomain=Discrete-time  UseExternalTs=off  SampleTime=-1  IntegratorMethod=Forward Euler  FilterMethod=Forward Euler  ControllerParametersSource=internal  P=controlParams.P_Z  I=controlParams.I_Z  UseKiTs=off  D=controlParams.D_Z  UseExternalDerivativeSource=off  N=controlParams.N_Z  UseFilter=on  TunerSelectOption=Transfer Function Based (PID Tuner App)  InitialConditionSource=internal  InitialConditionForIntegrator=0  InitialConditionForFilter=0  DifferentiatorICPrevScaledInput=0  ExternalReset=none  TrackingMode=off  Kt=1  LimitOutput=off  SatLimitsSource=internal  UpperSaturationLimit=inf  LowerSaturationLimit=-inf  LinearizeAsGain=on  AntiWindupMode=none  Kb=1  LimitIntegrator=off  UpperIntegratorSaturationLimit=inf  LowerIntegratorSaturationLimit=-inf  POutMin=[]  POutMax=[]  IOutMin=[]  IOutMax=[]  DOutMin=[]  DOutMax=[]  NOutMin=[]  NOutMax=[]  SumOutMin=[]  SumOutMax=[]  SaturationOutMin=[]  SaturationOutMax=[]  PParamMin=[]  PParamMax=[]  IParamMin=[]  IParamMax=[]  DParamMin=[]  DParamMax=[]  NParamMin=[]  NParamMax=[]  KbParamMin=[]  KbParamMax=[]  KtParamMin=[]  KtParamMax=[]  KbOutMin=[]  KbOutMax=[]  KtOutMin=[]  KtOutMax=[]  IntegratorOutMin=[]  IntegratorOutMax=[]  FilterOutMin=[]  FilterOutMax=[]  SumI1OutMin=[]  SumI1OutMax=[]  SumI2OutMin=[]  SumI2OutMax=[]  SumI3OutMin=[]  SumI3OutMax=[]  SumI4OutMin=[]  SumI4OutMax=[]  SumDOutMin=[]  SumDOutMax=[]  DifferentiatorOutMin=[]  DifferentiatorOutMax=[]  FilterDiffOutCoefMin=[]  FilterDiffOutCoefMax=[]  ReciprocalOutMin=[]  ReciprocalOutMax=[]  SumDenOutMin=[]  SumDenOutMax=[]  SumNumOutMin=[]  SumNumOutMax=[]  DivideOutMin=[]  DivideOutMax=[]  UdiffTsProdOutMin=[]  UdiffTsProdOutMax=[]  NTsProdOutMin=[]  NTsProdOutMax=[]  UintegralTsProdOutMin=[]  UintegralTsProdOutMax=[]  UngainTsProdOutMin=[]  UngainTsProdOutMax=[]  ClampingZeroOutDataTypeStr=Inherit: Inherit via back propagation  ClampingZeroOutMin=[]  ClampingZeroOutMax=[]  FilterDenConstantOutDataTypeStr=Inherit: Inherit via back propagation  FilterDenConstantOutMin=[]  FilterDenConstantOutMax=[]  PCopyOutDataTypeStr=Inherit: Inherit via back propagation  PCopyOutMin=[]  PCopyOutMax=[]  NCopyOutDataTypeStr=Inherit: Inherit via back propagation  NCopyOutMin=[]  NCopyOutMax=[]  IntegratorContinuousStateAttributes=''  IntegratorStateMustResolveToSignalObject=off  IntegratorRTWStateStorageClass=Auto  FilterContinuousStateAttributes=''  FilterStateMustResolveToSignalObject=off  FilterRTWStateStorageClass=Auto  ParallelPVariant=InternalParameters  IdealPVariant=Disabled  IVariant=Disabled  DVariant=Disabled  IntegratorVariant=Disabled  SatVariant=Disabled  AWVariant=Disabled  PCopyVariant=Disabled  TRVariant=Disabled  FdbkBlocksVariant=Forward  IdealPFdbkVariant=Disabled  SatFdbkVariant=Disabled  DerivativeFilterVariant=Disabled  NVariant=Disabled  NCopyVariant=Disabled_SignalSpec  FilterICVariant=Disabled  IntegratorICVariant=Disabled  ExternalResetVariant=Disabled  TRSumVariant=Passthrough  SumFdbkVariant=Disabled  SumVariant=Passthrough_P  TsampFilterVariant=InternalTs  TsampNgainVariant=Passthrough  TsampIntegralVariant=Disabled_SignalSpec  ExternalSaturationOutDataTypeStr=Inherit: Same as second input  DerivativeSourceVariant=Disabled  PreIntVariant=InternalPreInt
  Altitude rate controller : slpidlib/PID Controller  Controller=PD  Form=Parallel  TimeDomain=Discrete-time  UseExternalTs=off  SampleTime=-1  IntegratorMethod=Forward Euler  FilterMethod=Forward Euler  ControllerParametersSource=internal  P=controlParams.P_VZ  I=controlParams.I_VZ/10  UseKiTs=off  D=controlParams.D_VZ  UseExternalDerivativeSource=off  N=controlParams.N_VZ  UseFilter=on  TunerSelectOption=Transfer Function Based (PID Tuner App)  InitialConditionSource=internal  InitialConditionForIntegrator=0  InitialConditionForFilter=0  DifferentiatorICPrevScaledInput=0  ExternalReset=none  TrackingMode=off  Kt=1  LimitOutput=off  SatLimitsSource=internal  UpperSaturationLimit=inf  LowerSaturationLimit=-inf  LinearizeAsGain=on  AntiWindupMode=none  Kb=1  LimitIntegrator=off  UpperIntegratorSaturationLimit=inf  LowerIntegratorSaturationLimit=-inf  POutMin=[]  POutMax=[]  IOutMin=[]  IOutMax=[]  DOutMin=[]  DOutMax=[]  NOutMin=[]  NOutMax=[]  SumOutMin=[]  SumOutMax=[]  SaturationOutMin=[]  SaturationOutMax=[]  PParamMin=[]  PParamMax=[]  IParamMin=[]  IParamMax=[]  DParamMin=[]  DParamMax=[]  NParamMin=[]  NParamMax=[]  KbParamMin=[]  KbParamMax=[]  KtParamMin=[]  KtParamMax=[]  KbOutMin=[]  KbOutMax=[]  KtOutMin=[]  KtOutMax=[]  IntegratorOutMin=[]  IntegratorOutMax=[]  FilterOutMin=[]  FilterOutMax=[]  SumI1OutMin=[]  SumI1OutMax=[]  SumI2OutMin=[]  SumI2OutMax=[]  SumI3OutMin=[]  SumI3OutMax=[]  SumI4OutMin=[]  SumI4OutMax=[]  SumDOutMin=[]  SumDOutMax=[]  DifferentiatorOutMin=[]  DifferentiatorOutMax=[]  FilterDiffOutCoefMin=[]  FilterDiffOutCoefMax=[]  ReciprocalOutMin=[]  ReciprocalOutMax=[]  SumDenOutMin=[]  SumDenOutMax=[]  SumNumOutMin=[]  SumNumOutMax=[]  DivideOutMin=[]  DivideOutMax=[]  UdiffTsProdOutMin=[]  UdiffTsProdOutMax=[]  NTsProdOutMin=[]  NTsProdOutMax=[]  UintegralTsProdOutMin=[]  UintegralTsProdOutMax=[]  UngainTsProdOutMin=[]  UngainTsProdOutMax=[]  ClampingZeroOutDataTypeStr=Inherit: Inherit via back propagation  ClampingZeroOutMin=[]  ClampingZeroOutMax=[]  FilterDenConstantOutDataTypeStr=Inherit: Inherit via back propagation  FilterDenConstantOutMin=[]  FilterDenConstantOutMax=[]  PCopyOutDataTypeStr=Inherit: Inherit via back propagation  PCopyOutMin=[]  PCopyOutMax=[]  NCopyOutDataTypeStr=Inherit: Inherit via back propagation  NCopyOutMin=[]  NCopyOutMax=[]  IntegratorContinuousStateAttributes=''  IntegratorStateMustResolveToSignalObject=off  IntegratorRTWStateStorageClass=Auto  FilterContinuousStateAttributes=''  FilterStateMustResolveToSignalObject=off  FilterRTWStateStorageClass=Auto  ParallelPVariant=InternalParameters  IdealPVariant=Disabled  IVariant=Disabled  DVariant=InternalParameters  IntegratorVariant=Disabled  SatVariant=Disabled  AWVariant=Disabled  PCopyVariant=Disabled  TRVariant=Disabled  FdbkBlocksVariant=Forward  IdealPFdbkVariant=Disabled  SatFdbkVariant=Disabled  DerivativeFilterVariant=ForwardEulerFilter  NVariant=InternalParameters  NCopyVariant=Disabled  FilterICVariant=InternalICsFilter  IntegratorICVariant=Disabled  ExternalResetVariant=Disabled  TRSumVariant=Passthrough  SumFdbkVariant=Disabled  SumVariant=Sum_PD  TsampFilterVariant=InternalTs  TsampNgainVariant=Passthrough  TsampIntegralVariant=Disabled_SignalSpec  ExternalSaturationOutDataTypeStr=Inherit: Same as second input  DerivativeSourceVariant=ErrorSignal  PreIntVariant=InternalPreInt
  Bus Selector : BusSelector  OutputSignals=Xe,Ve
  Constant4 : Constant  Value=flightState.FixedWing
  Equal : RelationalOperator  Operator===  OutDataTypeStr=boolean  RndMeth=Simplest  InputSameDT=off
  NOT : Logic  Operator=NOT  IconShape=distinctive  AllPortsSameDT=off  OutDataTypeStr=boolean
  Rate Limiter : RateLimiter  FallingSlewLimit=-1000  SampleTimeMode=inherited
  Selector : Selector  InputPortWidth=3  IndexOptions=Index vector (dialog)  Indices=[3]  OutputSizes=1
  Selector1 : Selector  InputPortWidth=3  IndexOptions=Index vector (dialog)  Indices=[3]  OutputSizes=1
  Sum : Sum  Inputs=|+-
  Sum1 : Sum  Inputs=|++
  Switch : Switch  Criteria=u2 > Threshold  SaturateOnIntegerOverflow=off  InputSameDT=off
  Switch1 : Switch  Criteria=u2 > Threshold  SaturateOnIntegerOverflow=off  InputSameDT=off
  Triggered Subsystem : Subsystem  TreatAsAtomicUnit=on
  commanded thrust : Outport
  wires:
  Altitude rate controller/1 -> commanded thrust/1  "Output"
  Selector1/1 -> Sum1/2
  Sum/1 -> Altitude controller/1
  Switch1/1 -> Switch/1  "Output"
  Z ref/1 -> Switch1/3  "Manual"
  Equal/1 -> Switch1/2
  FlightMode/1 -> Equal/2
  Constant4/1 -> Equal/1
  Altitude controller/1 -> Sum1/1
  Alt signal condition/1(Z_out) -> Sum/2
  Rate Limiter/1 -> Sum/1
  Sum1/1 -> Altitude rate controller/1
  Bus Selector/2 -> Selector1/1  "<Ve>"
  Bus Selector/1 -> Selector/1  "<Xe>"
  Selector/1 -> Triggered Subsystem/1(AltHold), Alt signal condition/1(Z_in)
  Triggered Subsystem/1(Reference) -> Switch/3, Switch1/1  "Stable"
  NOT/1 -> Switch/2
  Switch/1 -> Rate Limiter/1  "Output"
  InTransition/1 -> Triggered Subsystem/Trigger, NOT/1
  States/1 -> Bus Selector/1
